simulink model "CEngDsT_DD"  (R2016b)
settings: configuration reference "CodeGenConfigSet" (kept outside this file)
values from neighbouring files (symbols this model uses):
  CEngDsT_tiMaxDefDeb_C = Calibration.Parameter    [init_CEngDsT_DD.m]
  CEngDsT_tiMaxOKDeb_C = Calibration.Parameter    [init_CEngDsT_DD.m]
  CEngDsT_tiMinDefDeb_C = Calibration.Parameter    [init_CEngDsT_DD.m]
  CEngDsT_tiMinOKDeb_C = Calibration.Parameter    [init_CEngDsT_DD.m]
  CEngDsT_tiPhysRngHiDefDeb_C = Calibration.Parameter    [init_CEngDsT_DD.m]
  CEngDsT_tiPhysRngHiOKDeb_C = Calibration.Parameter    [init_CEngDsT_DD.m]
  CEngDsT_tiPhysRngLoDefDeb_C = Calibration.Parameter    [init_CEngDsT_DD.m]
  CEngDsT_tiPhysRngLoOKDeb_C = Calibration.Parameter    [init_CEngDsT_DD.m]
  CEngDsT_tPhysRngMax_C = Calibration.Parameter    [init_CEngDsT_DD.m]
  CEngDsT_tPhysRngMin_C = Calibration.Parameter    [init_CEngDsT_DD.m]
  CEngDsT_tTransf_CUR = Calibration.Parameter    [init_CEngDsT_DD.m]
  CEngDsT_tTransf_CURX = Calibration.Parameter    [init_CEngDsT_DD.m]
  CEngDsT_uSRCMax_C = Calibration.Parameter    [init_CEngDsT_DD.m]
  CEngDsT_uSRCMin_C = Calibration.Parameter    [init_CEngDsT_DD.m]
undefined symbols (not defined in the file or in its folder): CEngDsT_DD_DT
libraries: CXLib x12
settings Model: Creator=Administrator  LastModifiedBy=wangrui
settings ConfigSetRef: SourceLocation=Base Workspace

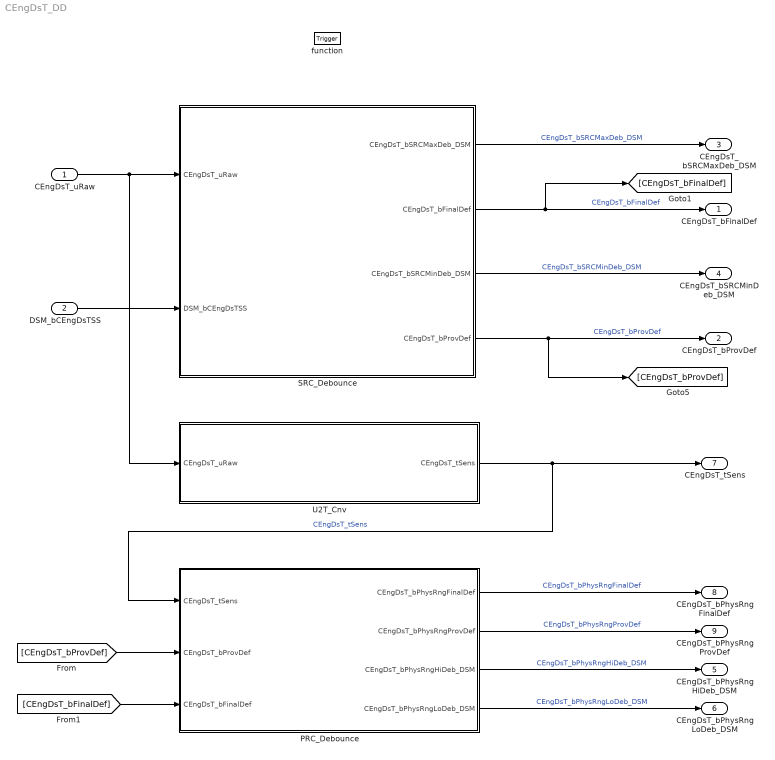
== system CEngDsT_DD ==
  CEngDsT_uRaw : Inport  Tag=mv  Description=Raw ADC value of downstream engine coolant temperature sensor signal  OutMin=0  OutMax=5000  OutDataTypeStr=Ad_mv
  DSM_bCEngDsTSS : Inport  Description=Status of FId_CEngDsTSS  Port=2  OutMin=0  OutMax=1  OutDataTypeStr=boolean
  function : TriggerPort  TriggerType=function-call  VariantControl=Variant
  PRC_Debounce : Subsystem
  SRC_Debounce : Subsystem
  U2T_Cnv : Subsystem
  CEngDsT_bFinalDef : Outport  Description=Status Sensor of the coolant temperature finally defect  OutMin=0  OutMax=1  OutDataTypeStr=boolean
  CEngDsT_bProvDef : Outport  Description=Status Sensor of the coolant temperature temporary defect  Port=2  OutMin=0  OutMax=1  OutDataTypeStr=boolean
  CEngDsT_bSRCMaxDeb_DSM : Outport  Description=status of CEngDsT_bSRCMaxDeb  Port=3  OutMin=0  OutMax=1  OutDataTypeStr=boolean
  CEngDsT_bSRCMinDeb_DSM : Outport  Description=status of CEngDsT_bSRCMinDeb  Port=4  OutMin=0  OutMax=1  OutDataTypeStr=boolean
  CEngDsT_bPhysRngHiDeb_DSM : Outport  Description=status of CEngDsT_bPhysRngHiDeb  Port=5  OutMin=0  OutMax=1  OutDataTypeStr=boolean
  CEngDsT_bPhysRngLoDeb_DSM : Outport  Description=status of CEngDsT_bPhysRngLoDeb  Port=6  OutMin=0  OutMax=1  OutDataTypeStr=boolean
  CEngDsT_tSens : Outport  Tag=deg  Description=Sensed engine coolant temperature  Port=7  OutMin=-200  OutMax=200  OutDataTypeStr=Temp_deg
  CEngDsT_bPhysRngFinalDef : Outport  Description=Status Sensor of the CEngDsT physical Signal range check finally defect  Port=8  OutMin=0  OutMax=1  OutDataTypeStr=boolean
  CEngDsT_bPhysRngProvDef : Outport  Description=Status Sensor of the CEngDsT physical Signal range check temporary defect  Port=9  OutMin=0  OutMax=1  OutDataTypeStr=boolean
  wires:
  CEngDsT_uRaw/1 -> SRC_Debounce/1(CEngDsT_uRaw), U2T_Cnv/1(CEngDsT_uRaw)
  DSM_bCEngDsTSS/1 -> SRC_Debounce/2(DSM_bCEngDsTSS)
  SRC_Debounce/1(CEngDsT_bSRCMaxDeb_DSM) -> CEngDsT_bSRCMaxDeb_DSM/1  "CEngDsT_bSRCMaxDeb_DSM"
  SRC_Debounce/2(CEngDsT_bFinalDef) -> CEngDsT_bFinalDef/1, [CEngDsT_bFinalDef]  "CEngDsT_bFinalDef"
  SRC_Debounce/3(CEngDsT_bSRCMinDeb_DSM) -> CEngDsT_bSRCMinDeb_DSM/1  "CEngDsT_bSRCMinDeb_DSM"
  SRC_Debounce/4(CEngDsT_bProvDef) -> CEngDsT_bProvDef/1, [CEngDsT_bProvDef]  "CEngDsT_bProvDef"
  U2T_Cnv/1(CEngDsT_tSens) -> CEngDsT_tSens/1, PRC_Debounce/1(CEngDsT_tSens)  "CEngDsT_tSens"
  PRC_Debounce/1(CEngDsT_bPhysRngFinalDef) -> CEngDsT_bPhysRngFinalDef/1  "CEngDsT_bPhysRngFinalDef"
  PRC_Debounce/2(CEngDsT_bPhysRngProvDef) -> CEngDsT_bPhysRngProvDef/1  "CEngDsT_bPhysRngProvDef"
  PRC_Debounce/3(CEngDsT_bPhysRngHiDeb_DSM) -> CEngDsT_bPhysRngHiDeb_DSM/1  "CEngDsT_bPhysRngHiDeb_DSM"
  PRC_Debounce/4(CEngDsT_bPhysRngLoDeb_DSM) -> CEngDsT_bPhysRngLoDeb_DSM/1  "CEngDsT_bPhysRngLoDeb_DSM"
  [CEngDsT_bProvDef] -> PRC_Debounce/2(CEngDsT_bProvDef)
  [CEngDsT_bFinalDef] -> PRC_Debounce/3(CEngDsT_bFinalDef)

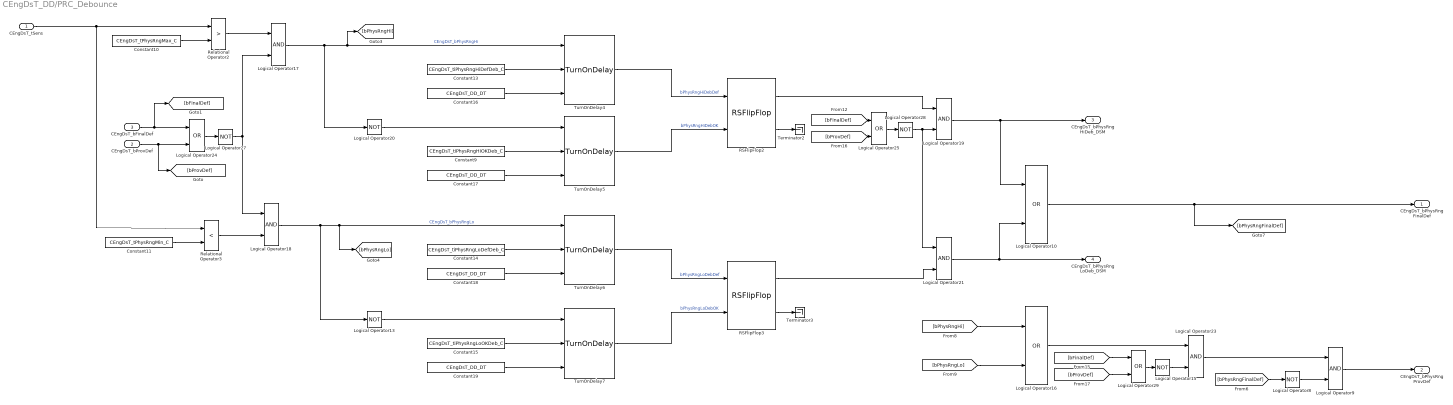
== system CEngDsT_DD/PRC_Debounce ==
  CEngDsT_tSens : Inport
  CEngDsT_bProvDef : Inport  Port=2
  CEngDsT_bFinalDef : Inport  Port=3
  Constant10 : Constant  Value=CEngDsT_tPhysRngMax_C
  Constant11 : Constant  Value=CEngDsT_tPhysRngMin_C
  Constant13 : Constant  Value=CEngDsT_tiPhysRngHiDefDeb_C
  Constant14 : Constant  Value=CEngDsT_tiPhysRngLoDefDeb_C
  Constant15 : Constant  Value=CEngDsT_tiPhysRngLoOKDeb_C
  Constant{16..19} (4 alike) : Constant  Value=CEngDsT_DD_DT  OutDataTypeStr=Inherit: Inherit via back propagation
  Constant9 : Constant  Value=CEngDsT_tiPhysRngHiOKDeb_C
  Logical Operator10 : Logic  Operator=OR  AllPortsSameDT=off  OutDataTypeStr=boolean
  Logical Operator{8,13,15,20,27..28} (6 alike) : Logic  Operator=NOT  AllPortsSameDT=off  OutDataTypeStr=boolean
  Logical Operator16 : Logic  Operator=OR  AllPortsSameDT=off  OutDataTypeStr=boolean
  Logical Operator{9,17..19,21,23} (6 alike) : Logic  AllPortsSameDT=off  OutDataTypeStr=boolean
  Logical Operator24 : Logic  RequirementInfo={} %GIDa_3e7d96dc_9b6a_4108_b1d0_1bc9d9c34b99  Operator=OR  OutDataTypeStr=boolean
  Logical Operator25 : Logic  RequirementInfo={} %GIDa_baaf25b8_17f6_4b56_9af5_8cf76abe6a51  Operator=OR  OutDataTypeStr=boolean
  Logical Operator29 : Logic  RequirementInfo={} %GIDa_14018441_c245_4cf6_873d_bb3a4539f13f  Operator=OR  OutDataTypeStr=boolean
  RSFlipFlop2 : CXLib/RSFlipFlop
  RSFlipFlop3 : CXLib/RSFlipFlop
  Relational Operator2 : RelationalOperator  Operator=>  OutDataTypeStr=boolean  RndMeth=Nearest  InputSameDT=on
  Relational Operator3 : RelationalOperator  Operator=<  OutDataTypeStr=boolean  RndMeth=Nearest  InputSameDT=on
  Terminator2 : Terminator
  Terminator3 : Terminator
  TurnOnDelay{4..7} (4 alike) : CXLib/TurnOnDelay
  CEngDsT_bPhysRngFinalDef : Outport  Tag=-  Description=Status Sensor of the coolant temperature physical Signal range check finally defect  OutMin=0  OutMax=1  OutDataTypeStr=boolean
  CEngDsT_bPhysRngProvDef : Outport  Tag=-  Description=Status Sensor of the coolant temperature physical Signal range check temporary defect  Port=2  OutMin=0  OutMax=1  OutDataTypeStr=boolean
  CEngDsT_bPhysRngHiDeb_DSM : Outport  Tag=-  Description=status of CEngDsT_bPhysRngHiDeb  Port=3  OutMin=0  OutMax=1  OutDataTypeStr=boolean
  CEngDsT_bPhysRngLoDeb_DSM : Outport  Tag=-  Description=status of CEngDsT_bPhysRngLoDeb  Port=4  OutMin=0  OutMax=1  OutDataTypeStr=boolean
  wires:
  CEngDsT_tSens/1 -> Relational Operator2/1, Relational Operator3/1
  Constant15/1 -> TurnOnDelay7/2
  TurnOnDelay7/1 -> RSFlipFlop3/2  "bPhysRngLoDebOK"
  Logical Operator13/1 -> TurnOnDelay7/1
  TurnOnDelay6/1 -> RSFlipFlop3/1  "bPhysRngLoDebDef"
  Logical Operator20/1 -> TurnOnDelay5/1
  TurnOnDelay4/1 -> RSFlipFlop2/1  "bPhysRngHiDebDef"
  Constant13/1 -> TurnOnDelay4/2
  Constant9/1 -> TurnOnDelay5/2
  Constant14/1 -> TurnOnDelay6/2
  TurnOnDelay5/1 -> RSFlipFlop2/2  "bPhysRngHiDebOK"
  RSFlipFlop2/1 -> Logical Operator19/1
  RSFlipFlop3/1 -> Logical Operator21/2
  Constant16/1 -> TurnOnDelay4/3
  Constant17/1 -> TurnOnDelay5/3
  Constant18/1 -> TurnOnDelay6/3
  Constant19/1 -> TurnOnDelay7/3
  Constant10/1 -> Relational Operator2/2
  Logical Operator17/1 -> [bPhysRngHi], TurnOnDelay4/1, Logical Operator20/1  "CEngDsT_bPhysRngHi"
  Constant11/1 -> Relational Operator3/2
  Logical Operator18/1 -> Logical Operator13/1, TurnOnDelay6/1, [bPhysRngLo]  "CEngDsT_bPhysRngLo"
  Logical Operator19/1 -> Logical Operator10/1, CEngDsT_bPhysRngHiDeb_DSM/1
  Logical Operator21/1 -> CEngDsT_bPhysRngLoDeb_DSM/1, Logical Operator10/2
  [bPhysRngHi] -> Logical Operator16/1
  [bPhysRngLo] -> Logical Operator16/2
  Relational Operator2/1 -> Logical Operator17/1
  Logical Operator24/1 -> Logical Operator27/1
  Logical Operator25/1 -> Logical Operator28/1
  Logical Operator16/1 -> Logical Operator23/1
  Logical Operator10/1 -> CEngDsT_bPhysRngFinalDef/1, [bPhysRngFinalDef]
  Logical Operator15/1 -> Logical Operator23/2
  Relational Operator3/1 -> Logical Operator18/2
  CEngDsT_bFinalDef/1 -> [bFinalDef], Logical Operator24/1
  CEngDsT_bProvDef/1 -> Logical Operator24/2, [bProvDef]
  [bFinalDef] -> Logical Operator25/1
  [bProvDef] -> Logical Operator25/2
  Logical Operator27/1 -> Logical Operator17/2, Logical Operator18/1
  Logical Operator28/1 -> Logical Operator21/1, Logical Operator19/2
  [bFinalDef] -> Logical Operator29/1
  [bProvDef] -> Logical Operator29/2
  Logical Operator29/1 -> Logical Operator15/1
  [bPhysRngFinalDef] -> Logical Operator8/1
  Logical Operator8/1 -> Logical Operator9/2
  Logical Operator23/1 -> Logical Operator9/1
  Logical Operator9/1 -> CEngDsT_bPhysRngProvDef/1
  RSFlipFlop3/2 -> Terminator3/1
  RSFlipFlop2/2 -> Terminator2/1

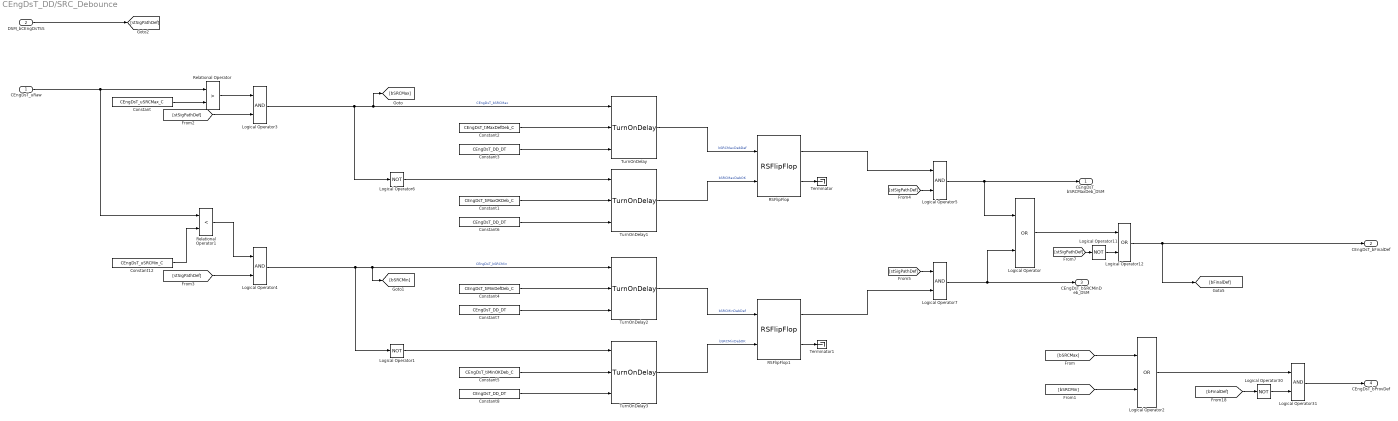
== system CEngDsT_DD/SRC_Debounce ==
  CEngDsT_uRaw : Inport  Tag=mv  Description=Raw ADC value of downstream engine coolant temperature sensor signal  OutMin=0  OutMax=5000  OutDataTypeStr=Ad_mv
  DSM_bCEngDsTSS : Inport  Tag=-  Description=Status of FId_CEngDsTSS  Port=2  OutMin=0  OutMax=1  OutDataTypeStr=boolean
  Constant : Constant  Value=CEngDsT_uSRCMax_C
  Constant1 : Constant  Value=CEngDsT_tiMaxOKDeb_C
  Constant12 : Constant  Value=CEngDsT_uSRCMin_C
  Constant2 : Constant  Value=CEngDsT_tiMaxDefDeb_C
  Constant{3,6..8} (4 alike) : Constant  Value=CEngDsT_DD_DT  OutDataTypeStr=Inherit: Inherit via back propagation
  Constant4 : Constant  Value=CEngDsT_tiMinDefDeb_C
  Constant5 : Constant  Value=CEngDsT_tiMinOKDeb_C
  Logical Operator : Logic  Operator=OR  AllPortsSameDT=off  OutDataTypeStr=boolean
  Logical Operator{1,6,11,30} (4 alike) : Logic  Operator=NOT  AllPortsSameDT=off  OutDataTypeStr=boolean
  Logical Operator12 : Logic  Operator=OR  AllPortsSameDT=off  OutDataTypeStr=boolean
  Logical Operator2 : Logic  Operator=OR  AllPortsSameDT=off  OutDataTypeStr=boolean
  Logical Operator{3..5,7,31} (5 alike) : Logic  AllPortsSameDT=off  OutDataTypeStr=boolean
  RSFlipFlop : CXLib/RSFlipFlop
  RSFlipFlop1 : CXLib/RSFlipFlop
  Relational Operator : RelationalOperator  Operator=>  OutDataTypeStr=boolean  RndMeth=Nearest  InputSameDT=on
  Relational Operator1 : RelationalOperator  Operator=<  OutDataTypeStr=boolean  RndMeth=Nearest  InputSameDT=on
  Terminator : Terminator
  Terminator1 : Terminator
  TurnOnDelay{,1..3} (4 alike) : CXLib/TurnOnDelay
  CEngDsT_bSRCMaxDeb_DSM : Outport  Tag=-  Description=status of CEngDsT_bSRCMaxDeb  OutMin=0  OutMax=1  OutDataTypeStr=boolean
  CEngDsT_bFinalDef : Outport  Tag=-  Description=Status Sensor of the coolant temperature finally defect  Port=2  OutMin=0  OutMax=1  OutDataTypeStr=boolean
  CEngDsT_bSRCMinDeb_DSM : Outport  Tag=-  Description=status of CEngDsT_bSRCMinDeb  Port=3  OutMin=0  OutMax=1  OutDataTypeStr=boolean
  CEngDsT_bProvDef : Outport  Tag=-  Description=Status Sensor of the coolant temperature temporary defect  Port=4  OutMin=0  OutMax=1  OutDataTypeStr=boolean
  wires:
  Relational Operator1/1 -> Logical Operator4/1
  [stSigPathDef] -> Logical Operator4/2
  [stSigPathDef] -> Logical Operator5/2
  [stSigPathDef] -> Logical Operator7/1
  CEngDsT_uRaw/1 -> Relational Operator1/1, Relational Operator/1
  [bFinalDef] -> Logical Operator30/1
  Logical Operator30/1 -> Logical Operator31/2
  Logical Operator2/1 -> Logical Operator31/1
  Logical Operator31/1 -> CEngDsT_bProvDef/1
  Logical Operator/1 -> Logical Operator12/1
  [stSigPathDef] -> Logical Operator11/1
  Logical Operator11/1 -> Logical Operator12/2
  Logical Operator12/1 -> CEngDsT_bFinalDef/1, [bFinalDef]
  RSFlipFlop1/1 -> Logical Operator7/2
  RSFlipFlop/1 -> Logical Operator5/1
  TurnOnDelay1/1 -> RSFlipFlop/2  "bSRCMaxDebOK"
  Constant4/1 -> TurnOnDelay2/2
  Constant1/1 -> TurnOnDelay1/2
  Constant2/1 -> TurnOnDelay/2
  TurnOnDelay/1 -> RSFlipFlop/1  "bSRCMaxDebDef"
  Logical Operator6/1 -> TurnOnDelay1/1
  TurnOnDelay2/1 -> RSFlipFlop1/1  "bSRCMinDebDef"
  Logical Operator1/1 -> TurnOnDelay3/1
  TurnOnDelay3/1 -> RSFlipFlop1/2  "bSRCMinDebOK"
  Constant5/1 -> TurnOnDelay3/2
  RSFlipFlop/2 -> Terminator/1
  RSFlipFlop1/2 -> Terminator1/1
  Constant3/1 -> TurnOnDelay/3
  Constant6/1 -> TurnOnDelay1/3
  Constant7/1 -> TurnOnDelay2/3
  Constant8/1 -> TurnOnDelay3/3
  Constant/1 -> Relational Operator/2
  Logical Operator3/1 -> Logical Operator6/1, TurnOnDelay/1, [bSRCMax]  "CEngDsT_bSRCMax"
  Constant12/1 -> Relational Operator1/2
  Logical Operator4/1 -> Logical Operator1/1, TurnOnDelay2/1, [bSRCMin]  "CEngDsT_bSRCMin"
  Logical Operator5/1 -> CEngDsT_bSRCMaxDeb_DSM/1, Logical Operator/1
  Logical Operator7/1 -> CEngDsT_bSRCMinDeb_DSM/1, Logical Operator/2
  [bSRCMax] -> Logical Operator2/1
  [bSRCMin] -> Logical Operator2/2
  DSM_bCEngDsTSS/1 -> [stSigPathDef]
  Relational Operator/1 -> Logical Operator3/1
  [stSigPathDef] -> Logical Operator3/2

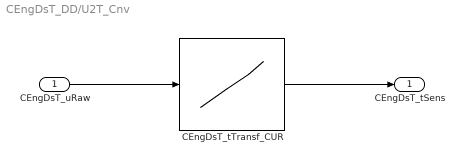
== system CEngDsT_DD/U2T_Cnv ==
  CEngDsT_uRaw : Inport  Tag=mv  Description=Raw ADC value of downstream engine coolant temperature sensor signal  OutMin=0  OutMax=5000  OutDataTypeStr=Ad_mv
  CEngDsT_tTransf_CUR : Lookup_n-D  RequirementInfo={} %GIDa_d4b8d1fd_3084_4373_a11d_5b41be8e7285  DialogController=Simulink.DDGSource  NumberOfTableDimensions=1  BreakpointsForDimension1=CEngDsT_tTransf_CURX  BreakpointsForDimension2=CEngDsT_tTransf_CURX  IndexSearchMethod=Linear search  BeginIndexSearchUsingPreviousIndexResult=on  Table=CEngDsT_tTransf_CUR  ExtrapMethod=Clip  UseLastTableValue=on  InternalRulePriority=Speed  OutDataTypeStr=Inherit: Inherit via back propagation  SaturateOnIntegerOverflow=on
  CEngDsT_tSens : Outport  Tag=deg  Description=Sensed engine coolant temperature  OutMin=-50  OutMax=150  OutDataTypeStr=Temp_deg
  wires:
  CEngDsT_uRaw/1 -> CEngDsT_tTransf_CUR/1
  CEngDsT_tTransf_CUR/1 -> CEngDsT_tSens/1
